simulink model "FluxModel2015a_verify_Q_zhixin"  (R2020b)
settings: Solver=VariableStepAuto  StartTime=0.0  StopTime=0.3  FixedStep=Ts  RelTol=1e-3  EnableMultiTasking=on
model workspace (MAT data in the model file):
  MOVE = Simulink.Parameter
  MOVE.Value = 1
  MOVE.DataType = 'boolean'
  MOVE.Dimensions = [1 1]
  STOP = Simulink.Parameter
  STOP.Value = 0
  STOP.DataType = 'boolean'
  STOP.Dimensions = [1 1]
  thres = Simulink.Parameter
  thres.Value = 0.1
  thres.DataType = 'double'
  thres.Dimensions = [1 1]
values from neighbouring files (symbols this model uses):
  AngleEncoderEn = 1    [parameters.m]
  AngleSpdClosedLoopEnable = 0.0    (= 0)    [parameters.m]
  CurrentLoopMax = Q14*1.2    (= 19660.8)    [parameters.m]
  EstOutMax_Speed_Q = Q14*1.2    (= 19660.8)    [parameters.m]
  Factor1 = Q15*Ts*Rb/Lq_realvalue    [parameters.m]
  Factor2 = Q15*Ts*Rs_realvalue/Lq_realvalue    (= 16990.2962963)    [parameters.m]
  fieldweaken_Max = 0    [parameters.m]
  fieldweaken_Min = -0.5*Q14    (= -8192)    [parameters.m]
  FieldWeakenEn = 0    [parameters.m]
  fluxF = Lam_realvalue/fluxB    [parameters.m]
  fluxF_Q14 = Q14*fluxF    [parameters.m]
  Friction = 0.003    [parameters.m]
  Ib = sqrt(2)*In    [parameters.m]
  Id_Ki = Q14*CurrentLoopBandwidth*Rs    [parameters.m]
  Id_Kp = Q14*CurrentLoopBandwidth*Ld    [parameters.m]
  IFCurrDecreased = 1    [parameters.m]
  IFCurrStart = 8    [parameters.m]
  IFCurrTarget = 5    [parameters.m]
  IFIdref = 0    [parameters.m]
  initial_degree = 0    [parameters.m]
  Iq_Ki = Q14*CurrentLoopBandwidth*Rs    [parameters.m]
  Iq_Kp = Q14*CurrentLoopBandwidth*Lq    [parameters.m]
  J_realvalue = 2.47e-4    (= 0.000247)    [parameters.m]
  KI_fieldweaken = 0.1*Q14    (= 1638.4)    [parameters.m]
  KP_fieldweaken = 1.0*Q14    (= 16384)    [parameters.m]
  LamObserverGain_Q = Q15*LamObserverGain    (= 13106.8)    [parameters.m]
  Ld = Ld_realvalue/Lb    [parameters.m]
  Ld_Q14 = Q14*Ld_realvalue/Lb    [parameters.m]
  Ld_realvalue = 2.7e-3    (= 0.0027)    [parameters.m]
  LowPassFilterBandWidth_Emf_Q = Q14*LowPassFilterBandWidth_Emf    (= 1445.64705882)    [parameters.m]
  LowPassFilterCoeff_Emf = Q15*(1/(1+LowPassFilterBandWidth_Emf*TsPu))    (= 31292.3812732)    [parameters.m]
  LowPassFilterCoeff_Spd = Q15*(1/(1+LowPassFilterBandWidth_Speed*SpeedloopTs/tb))    (= 20123.2126159)    [parameters.m]
  Lq = Lq_realvalue/Lb    [parameters.m]
  Lq_Q14 = Q14*Lq_realvalue/Lb    [parameters.m]
  Lq_realvalue = 2.7e-3    (= 0.0027)    [parameters.m]
  MOVE = 1    [parameters.m]
  Np = 1    [parameters.m]
  Omega0_Q = Q14*Omega0    (= 6553.6)    [parameters.m]
  OverModulationEn = 0    [parameters.m]
  PLL_KI = Q14*PLL_Bandwidth*PLL_Bandwidth    (= 56.6920415225)    [parameters.m]
  PLL_KP = Q14*2*PLL_Bandwidth    (= 1927.52941176)    [parameters.m]
  PLL_OUTMax_W = Q14*1.2    (= 19660.8)    [parameters.m]
  PWM_Period = 1000    [parameters.m]
  Q14 = 16384    [parameters.m]
  Q15 = 32767    [parameters.m]
  Q16 = 65535    [parameters.m]
  Rs = Rs_realvalue/Rb    [parameters.m]
  Rs_Q14 = Q14*Rs_realvalue/Rb    [parameters.m]
  Rs_realvalue = 28    [parameters.m]
  SecondOverMod = 0    [parameters.m]
  SMO_Gain = Q14*0.85    (= 13926.4)    [parameters.m]
  SMO_I_ERROR = Q14*0.05    (= 819.2)    [parameters.m]
  SpdClosedLoopEnable = 0.0    (= 0)    [parameters.m]
  Speed_Ki = Q14*SpeedLoopBandwidth    (= 481.882352941)    [parameters.m]
  Speed_Kp = Q14*SpeedLoopBandwidth*JPu/fluxF    [parameters.m]
  SpeedIncreased = 0.1*Wb    (= 1068.14150222)    [parameters.m]
  SpeedloopTs = 1/SpeedloopFrequency    (= 0.001)    [parameters.m]
  Speedn = 60*fn/Np    (= 102000)    [parameters.m]
  SpeedOutmax = 1.2*Q14    (= 19660.8)    [parameters.m]
  SpeedSwitch = 0.6*Wb    (= 6408.84901332)    [parameters.m]
  SpeedTarget = 0.8*Wb    (= 8545.13201776)    [parameters.m]
  STOP = 0    [parameters.m]
  SVCM_GAIN_Q = Q15*SVCM_GAIN    (= 26213.6)    [parameters.m]
  tb = 1/Wb    (= 9.36205547599e-05)    [parameters.m]
  Tf = 0    [parameters.m]
  thres = 0.1    [parameters.m]
  Tn = 0.012    [parameters.m]
  Ts = 1/SwitchFrequency    (= 5e-05)    [parameters.m]
  TsPu = Ts/tb    (= 0.53407075111)    [parameters.m]
  Vb = Vdc/sqrt(3)    [parameters.m]
  Vdc = sqrt(2)*Un    [parameters.m]
  Wb = 2*pi*fn    (= 10681.4150222)    [parameters.m]
  ZeroSeqInjectEn = 0.0    (= 0)    [parameters.m]
undefined symbols (not defined in the file or in its folder): DiscIntNeverNeededParam, EstOutMax_Theta, magnitude, sigbuilder_block
libraries: simulink x9, powerlib x5, mcbutilslib x1
(part 1 of 3)
settings Model: OrderedModelArguments=off  Creator=Administrator  LastModifiedBy=wangdi
settings DataIOCC: LimitDataPoints=on  SaveFormat=Array  ReturnWorkspaceOutputs=off
settings OptimizationCC: DefaultParameterBehavior=Inlined  DefaultUnderspecifiedDataType=single  EnhancedBackFolding=on  PassReuseOutputArgsAs=Individual arguments  ExpressionDepthLimit=2147483647  ZeroExternalMemoryAtStartup=off  ZeroInternalMemoryAtStartup=off  InitFltsAndDblsToZero=on  OptimizeBlockOrder=speed  DifferentSizesBufferReuse=on  OptimizationCustomize=off  EfficientTunableParamExpr=on
settings DebuggingCC: SaveWithParameterizedLinksMsg=none  UnderspecifiedInitializationDetection=Classic  MergeDetectMultiDrivingBlocksExec=none  SolverPrmCheckMsg=warning  ParameterTunabilityLossMsg=error  FcnCallInpInsideContextMsg=warning  StateNameClashWarn=warning  SFUnexpectedBacktrackingDiag=warning  SFNoUnconditionalDefaultTransitionDiag=warning  SFExecutionAtInitializationDiag=none  ArithmeticOperatorsInVariantConditions=warning
settings HardwareCC: ProdBitPerPointer=32  ProdBitPerSizeT=32  ProdBitPerPtrDiffT=32  ProdLargestAtomicFloat=None  ProdIntDivRoundTo=Undefined  ProdEndianess=Unspecified  ProdWordSize=32  ProdHWDeviceType=32-bit Generic
settings ModelReferenceCC: PropagateSignalLabelsOutOfModel=off
settings SFSimCC: SimUseLocalCustomCode=off  SimParseCustomCode=off  MATLABDynamicMemAlloc=off  CustomCodeUndefinedFunction=UseInterfaceOnly
settings RTWCC: Description=Embedded Coder  SystemTargetFile=ert.tlc  TemplateMakefile=ert_default_tmf  RTWUseLocalCustomCode=off
settings CodeAppCC: ForceParamTrailComments=on  IgnoreCustomStorageClasses=off  OperatorAnnotations=on  SimulinkDataObjDesc=on  SFDataObjDesc=on  InsertBlockDesc=on
settings ERTTargetCC: GenerateSampleERTMain=on  InlinedParameterPlacement=NonHierarchical  ERTCustomFileTemplate=example_file_process.tlc
settings ConfigComp: CovMetricSettings=dw  CovSaveCumulativeToWorkspaceVar=on  CovSaveSingleToWorkspaceVar=on  CovExternalEMLEnable=off
settings SimscapeCC: SimscapeNormalizeSystem=off

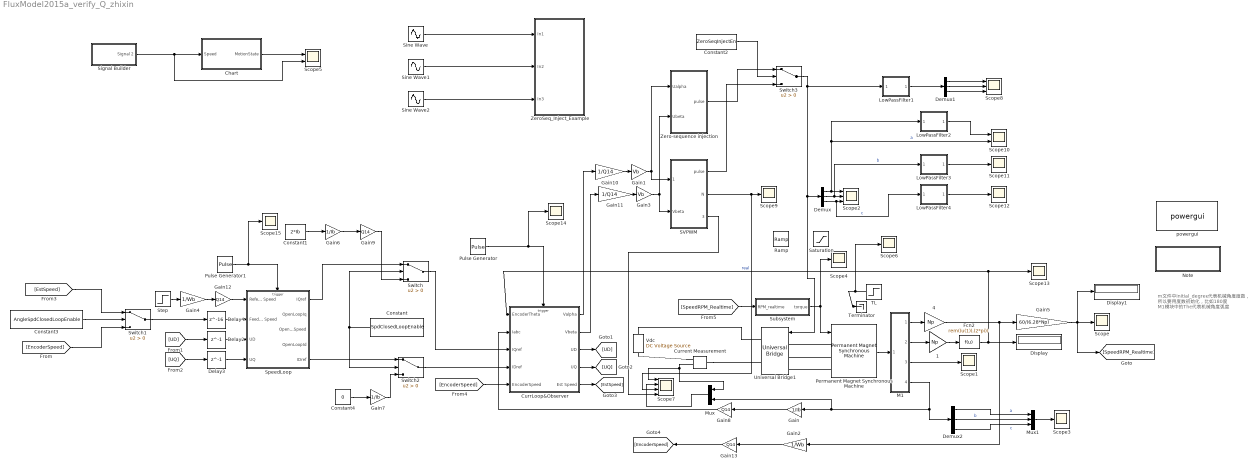
== system FluxModel2015a_verify_Q_zhixin ==
  note: m文件中initial_degree代表机械角度度数，
      | 所以要用度数初始化，比如180度
      | M1模块中的The代表机械角度弧度
  1 : Gain  Gain=Np
  4 : Gain  Gain=Np
  Chart : Stateflow chart  TreatAsAtomicUnit=on
  Constant : Constant  Value=SpdClosedLoopEnable
  Constant1 : Constant  Value=2*Ib
  Constant2 : Constant  Value=ZeroSeqInjectEn
  Constant3 : Constant  Value=AngleSpdClosedLoopEnable
  Constant4 : Constant  Value=0
  CurrLoop&Observer : Subsystem
  Current Measurement : powerlib/Measurements/Current Measurement  PhasorSimulation=off  OutputType=Complex  PSBequivalent=0
  Delay2 : Delay  DelayLength=1
  Delay3 : Delay  DelayLength=1
  Delay4 : Delay  DelayLength=16
  Demux : Demux  Outputs=3
  Demux1 : Demux  Outputs=3
  Demux2 : Demux  Outputs=3
  Display : Display
  Display1 : Display
  Fcn2 : Fcn  Expr=rem((u(1)),(2*pi))
  Gain : Gain  Gain=1/Ib
  Gain1 : Gain  Gain=Vb
  Gain10 : Gain  Gain=1/Q14
  Gain11 : Gain  Gain=1/Q14
  Gain{8..9,12..13} (4 alike) : Gain  Gain=Q14
  Gain2 : Gain  Gain=1/Wb
  Gain3 : Gain  Gain=Vb
  Gain4 : Gain  Gain=1/Wb
  Gain5 : Gain  Gain=60/(6.28*Np)
  Gain6 : Gain  Gain=1/Ib
  Gain7 : Gain  Gain=1/Ib
  LowPassFilter1 : Subsystem
  LowPassFilter2 : Subsystem
  LowPassFilter3 : Subsystem
  LowPassFilter4 : Subsystem
  M1 : Subsystem
  Mux : Mux  Inputs=2
  Mux1 : Mux  Inputs=3
  Note : Subsystem
  Permanent Magnet Synchronous Machine : powerlib/Machines/Permanent Magnet Synchronous Machine  NbPhases=3  FluxDistribution=Sinusoidal  RotorType=Salient-pole  MechanicalLoad=Torque Tm  PresetModel=No  ShowDetailedParameters=on  MeasurementBus=off  Resistance=Rs_realvalue  Inductance=8.5e-3  dqInductances=[Ld_realvalue, Lq_realvalue]  La=0.000835  MachineConstant=Flux linkage established by magnets (V.s)  Flux=Lam_realvalue  VoltageCst=11.7365  TorqueCst=0.09706  Flat=120  Mechanical=[J_realvalue Friction Np Tf]  PolePairs=Np  InitialConditions=[0,initial_degree, 0,0]  InitialConditions5ph=[0 0 0 0 0 0]  RefAngle=Aligned with phase A axis (original Park)  IterativeDiscreteModel=Trapezoidal non iterative  TsBlock=-1  TsPowergui=0
  Pulse Generator : DiscretePulseGenerator  PulseType=Time based  Period=Ts  PulseWidth=50
  Pulse Generator1 : DiscretePulseGenerator  PulseType=Time based  Period=SpeedloopTs  PulseWidth=50
  Ramp : simulink/Sources/Ramp  slope=5  start=0  InitialOutput=0
  SVPWM : Subsystem
  Saturation : Saturate  UpperLimit=0.2  LowerLimit=-0.2
  Scope{,1,3..4,6,9,11..15} (11 alike) : Scope
  Scope10 : Scope  NumInputPorts=2
  Scope2 : Scope  NumInputPorts=3
  Scope5 : Scope  NumInputPorts=2
  Scope7 : Scope  NumInputPorts=4
  Scope8 : Scope  NumInputPorts=3
  Signal Builder : Subsystem  Tag=STV Subsys  LoadFcn=sigbuilder_block('load');  StartFcn=sigbuilder_block('start');  StopFcn=sigbuilder_block('stop');  ClipboardFcn=sigbuilder_block('clipboard');  mask(Sigbuilder block){tuvar=[0:10]}
      mask help: Simulink:masks:SigbuilderBlock_MD
      mask init:
      | if ~strcmp(get_param(bdroot(gcbh),'SimulationStatus'),'stopped') tuvar = sigbuilder_block('maskInit'); end
      settings: CopyFcn=sigbuilder_block('copy');  DeleteFcn=sigbuilder_block('delete');  ModelCloseFcn=sigbuilder_block('modelClose');  PreSaveFcn=sigbuilder_block('preSave');  PauseFcn=sigbuilder_block('pause');  ContinueFcn=sigbuilder_block('continue');  NameChangeFcn=sigbuilder_block('namechange');  OpenFcn=sigbuilder_block('open',[1951.5 -31.5 550.5 326 ]);  CloseFcn=sigbuilder_block('close');
      mask Display: plot(0, 0, 100, 100,[2, 2, 32, 32, 2], [68, 8, 8, 68, 68],[32, 2], [38, 38], [32, 19, 2],[53, 60, 44], [32, 17, 17, 2],[16, 16, 31, 31]);txt = getActiveGroup(gcbh);text(2, 100, txt,'verticalAlignment', 'top');
  Sine Wave : Sin  Frequency=10*6.28
  Sine Wave1 : Sin  Frequency=10*6.28  Phase=2*pi/3
  Sine Wave2 : Sin  Frequency=10*6.28  Phase=4*pi/3
  SpeedLoop : Subsystem
  Step : Step  Time=0  After=1.5*Wb  SampleTime=0
  Subsystem : Subsystem
  Switch{,1..3} (4 alike) : Switch  Criteria=u2 > Threshold
  TL : Step  Time=0  Before=1  After=2.88  SampleTime=0
  Terminator : Terminator
  Universal Bridge1 : powerlib/Power Electronics/Universal Bridge  Arms=3  SnubberResistance=1e5  SnubberCapacitance=inf  Device=IGBT / Diodes  Ron=1e-3  Lon=0  ForwardVoltages="[  0  0  ]"  ForwardVoltage=0  GTOparameters=[ 10e-6 , 20e-6 ]  IGBTparameters=[ 1e-6 , 2e-6 ]  Measurements=None  Measurements_2=None  converterType=Rectifier
  Vdc : powerlib/Electrical Sources/DC Voltage Source  Amplitude=Vdc  Measurements=None
  Zero-sequence injection : Subsystem
  ZeroSeq_Inject_Example : Subsystem
  powergui : powerlib/powergui  SimulationMode=Discrete  SampleTime=Ts/100  frequency=60  Iterations=50  frequencyindice=0  Pbase=100e6  ErrMax=1e-4  UnitsV=kV  UnitsW=MW  buscounter=0  FunctionMessages=off  echomessages=off  EnableUseOfTLC=off  CurrentSourceSwitches=off  DisableSnubberDevices=off  DisableRonSwitches=off  DisableVfSwitches=off  DisplayEquations=off  AutomaticDiscreteSolvers=off  SolverType=Tustin/Backward Euler (TBE)  Interpol=off  ExternalGateDelay=off  methode=off  Ts=0  x0status=blocks  SPID=off  SwTol=0  HookPort=off  NonlinearTolerance=1e-4  nMaxIteration=100  ContinueOnMaxIteration=off  RestoreLinks=warning  ResistiveCurrentMeasurement=off  Frange=[0:2:500]  Ylog=off  Xlog=on  ShowGrid=off  save=off  variable=ZData  structure=0  ZoomFFT=off  StartTime=0.0  cycles=1  DisplayStyle=1  fundamental=60  FreqAxis=off  MaxFrequency=1000  frequencyindicesteady=1  RmsSteady=1  display=off
  wires:
  M1/4(Iabc) -> Demux2/1, Mux/2, Gain/1
  M1/2(The) -> 1/1
  Permanent Magnet Synchronous Machine/1 -> M1/1(In1)
  1/1 -> Fcn2/1
  M1/1(wm) -> 4/1
  M1/3(Te) -> Scope1/1
  4/1 -> Gain5/1, Gain2/1
  Fcn2/1 -> Display/1, CurrLoop&Observer/1(EncoderTheta), Scope13/1  "real"
  Pulse Generator/1 -> Scope14/1, CurrLoop&Observer/Trigger
  Demux2/1 -> Mux1/1  "a"
  Demux2/2 -> Mux1/2  "b"
  Demux2/3 -> Mux1/3  "c"
  Demux/1 -> Scope10/2, LowPassFilter2/1(Input), Scope2/1  "a"
  Demux/2 -> LowPassFilter3/1(Input), Scope2/2  "b"
  Demux/3 -> LowPassFilter4/1(Input), Scope2/3  "c"
  TL/1 -> Scope6/1, Terminator/1
  Gain/1 -> Gain8/1
  Current Measurement/1 -> Mux/1, Scope7/1
  Mux/1 -> Scope7/2
  SVPWM/2(N) -> Scope7/3, Scope9/1
  SVPWM/3(Output) -> Scope7/4
  LowPassFilter1/1(Output) -> Demux1/1
  Demux1/1 -> Scope8/1
  Demux1/2 -> Scope8/2
  Demux1/3 -> Scope8/3
  LowPassFilter2/1(Output) -> Scope10/1
  LowPassFilter3/1(Output) -> Scope11/1
  LowPassFilter4/1(Output) -> Scope12/1
  Mux1/1 -> Scope3/1
  Gain5/1 -> [SpeedRPM_Realtime], Display1/1, Scope/1
  Pulse Generator1/1 -> Scope15/1, SpeedLoop/Trigger
  Gain6/1 -> Gain9/1
  Constant1/1 -> Gain6/1
  CurrLoop&Observer/3(UD) -> [UD]
  CurrLoop&Observer/4(UQ) -> [UQ]
  [UD] -> Delay2/1
  [UQ] -> Delay3/1
  SpeedLoop/1(IQref) -> Switch/1
  Step/1 -> Gain4/1
  CurrLoop&Observer/5(Est Speed) -> [EstSpeed]
  Constant3/1 -> Switch1/2
  [EstSpeed] -> Switch1/1
  [EncoderSpeed] -> Switch1/3
  [EncoderSpeed] -> CurrLoop&Observer/5(EncoderSpeed)
  Delay2/1 -> SpeedLoop/3(UD)
  Delay3/1 -> SpeedLoop/4(UQ)
  Delay4/1 -> SpeedLoop/2(Feedback Speed)
  Signal Builder/1(Signal 2) -> Scope5/2, Chart/1(Speed)
  Chart/1(MotionState) -> Scope5/1
  Constant/1 -> Switch2/2, Switch/2
  Constant4/1 -> Gain7/1
  Gain7/1 -> Switch2/3
  Gain8/1 -> CurrLoop&Observer/2(Iabc)
  Gain9/1 -> Switch/3
  Gain10/1 -> Gain1/1
  Gain11/1 -> Gain3/1
  Gain4/1 -> Gain12/1
  Gain2/1 -> Gain13/1
  Switch/1 -> CurrLoop&Observer/3(IQref)
  Switch2/1 -> CurrLoop&Observer/4(IDref)
  Switch1/1 -> Delay4/1
  Gain12/1 -> SpeedLoop/1(Reference Speed)
  Gain13/1 -> [EncoderSpeed]
  SpeedLoop/5(IDref) -> Switch2/1
  CurrLoop&Observer/1(Valpha) -> Gain10/1
  CurrLoop&Observer/2(Vbeta) -> Gain11/1
  Subsystem/1(torque) -> Permanent Magnet Synchronous Machine/1, Scope4/1
  [SpeedRPM_Realtime] -> Subsystem/1(RPM_realtime)
  Gain1/1 -> Zero-sequence injection/1(Ualpha), SVPWM/1(Valpha)
  Gain3/1 -> SVPWM/2(Vbeta), Zero-sequence injection/2(Ubeta)
  Constant2/1 -> Switch3/2
  Zero-sequence injection/1(pulse) -> Switch3/1
  SVPWM/1(pulse) -> Switch3/3
  Switch3/1 -> Demux/1, Universal Bridge1/1, LowPassFilter1/1(Input)
  Sine Wave/1 -> ZeroSeq_Inject_Example/1(In1)
  Sine Wave1/1 -> ZeroSeq_Inject_Example/2(In2)
  Sine Wave2/1 -> ZeroSeq_Inject_Example/3(In3)
  connections:
  Permanent Magnet Synchronous Machine/LConn3 -- Universal Bridge1/LConn3
  Vdc/RConn1 -- Universal Bridge1/RConn1
  Permanent Magnet Synchronous Machine/LConn1 -- Universal Bridge1/LConn1
  Permanent Magnet Synchronous Machine/LConn2 -- Universal Bridge1/LConn2
  Current Measurement/LConn1 -- Universal Bridge1/RConn2
  Current Measurement/RConn1 -- Vdc/LConn1

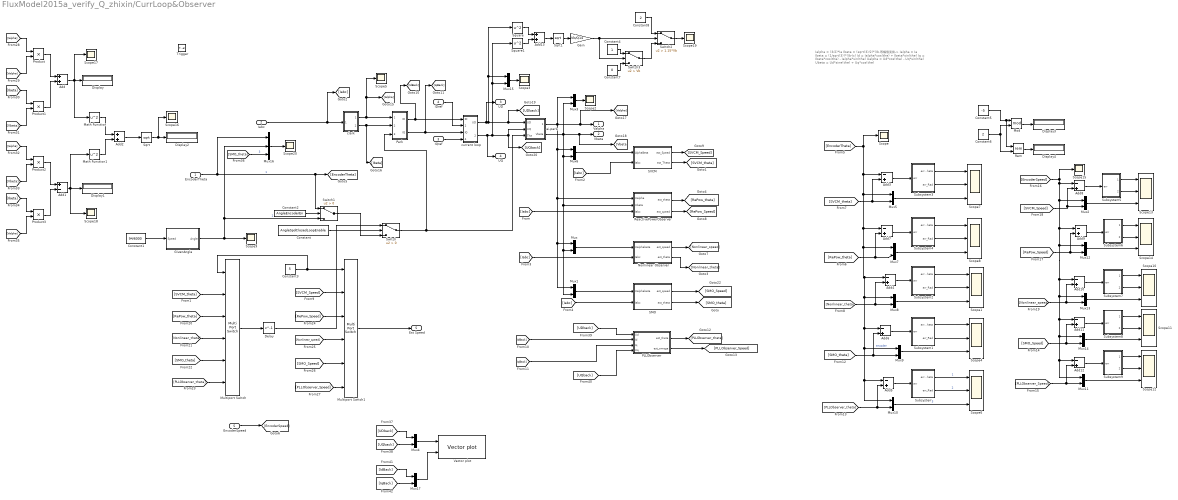
== system FluxModel2015a_verify_Q_zhixin/CurrLoop&Observer ==
  note: Ialpha = (3/2)*Ia
      | Ibeta = (sqrt(3)/2)*(Ib-Ic)
      | 等幅值变换->
      | Ialpha = Ia
      | Ibeta = (1/sqrt(3))*(Ib-Ic)
      |
      | Id = Ialpha*cos(the) + Ibeta*sin(the)
      | Iq = Ibeta*cos(the) - Ialpha*sin(the)
      |
      | Ualpha = Ud*cos(the) - Uq*sin(the)
      | Ubeta = Ud*sine(the) + Uq*cos(the)
  EncoderTheta : Inport
  Iabc : Inport  Port=2
  IQref : Inport  Port=3
  IDref : Inport  Port=4
  EncoderSpeed : Inport  Port=5
  Trigger : TriggerPort  VariantControl=(inherit)
  Add : Sum
  Add1 : Sum  Inputs=+-
  Add{3..12} (10 alike) : Sum  Inputs=-+
  Add13 : Sum
  Add2 : Sum
  Constant : Constant  Value=AngleSpdClosedLoopEnable
  Constant1 : Constant  Value=94/6000
  Constant2 : Constant  Value=AngleEncoderEn
  Constant3 : Constant  Value=5
  Constant4 : Constant
  Constant5 : Constant  Value=-5
  Constant6 : Constant  Value=2
  Constant7 : Constant  Value=0
  Constant8 : Constant  Value=2
  Delay : Delay  DelayLength=1
  Display{,1..4} (5 alike) : Display
  Gain : Gain  Gain=Vb/Q14
  GivenAngle : Subsystem
  Math Function : Math  Operator=square  SaturateOnIntegerOverflow=on
  Math Function1 : Math  Operator=square  SaturateOnIntegerOverflow=on
  Mod : Math  Operator=mod  SaturateOnIntegerOverflow=on
  Multiport Switch : MultiPortSwitch  Inputs=5
  Multiport Switch1 : MultiPortSwitch  Inputs=5
  Mux{,1..15,17} (17 alike) : Mux  Inputs=2
  Mux16 : Mux  Inputs=3
  Nonlinear Observer : Subsystem
  PLLObserver : Subsystem
  Park : Subsystem
  Product{,1..3} (4 alike) : Product
  ReactivePowerObserver : Subsystem
  Rem : Math  Operator=rem  SaturateOnIntegerOverflow=on
  SMO : Subsystem
  SVCM : Subsystem
  Scope{,2..3,5,9,15..20} (11 alike) : Scope
  Scope{1,4,6..8,10..14} (10 alike) : Scope  NumInputPorts=3
  Sqrt : Sqrt  SaturateOnIntegerOverflow=on
  Sqrt1 : Sqrt  SaturateOnIntegerOverflow=on
  Square : Math  Operator=square  SaturateOnIntegerOverflow=on
  Square1 : Math  Operator=square  SaturateOnIntegerOverflow=on
  Subsystem : Subsystem
  Subsystem1 : Subsystem
  Subsystem2 : Subsystem
  Subsystem3 : Subsystem
  Subsystem4 : Subsystem
  Subsystem5 : Subsystem
  Subsystem6 : Subsystem
  Subsystem7 : Subsystem
  Subsystem8 : Subsystem
  Subsystem9 : Subsystem
  Switch : Switch  Criteria=u2 > Threshold
  Switch1 : Switch  Criteria=u2 > Threshold
  Switch2 : Switch  Criteria=u2 > Threshold  Threshold=1.15*Vb
  Switch3 : Switch  Criteria=u2 > Threshold  Threshold=Vb
  Vector plot : mcbutilslib/Vector plot  InputSignals=Vdq Idq  ReferenceFrame=Rotating Reference Frame  axisAlign=D-axis  thetaUnits=Radians  angleUnits=Radians  OpenFigAtSimStart=on  debugEnable=0
      settings: SourceProductBaseCode=MT
  ai-park : Subsystem
  clark : Subsystem
  current loop : Subsystem
  Valpha : Outport
  Vbeta : Outport  Port=2
  UD : Outport  Port=3
  UQ : Outport  Port=4
  Est Speed : Outport  Port=5
  wires:
  Iabc/1 -> [Iabc], clark/1(Iabc)
  Park/1(ID) -> current loop/1(ID), [IdBack]
  Park/2(IQ) -> current loop/3(IQ), [IqBack]
  Mux3/1 -> Scope2/1
  EncoderTheta/1 -> Mux16/1, Switch1/1, [EncoderTheta]  "1"
  ai-park/1(Valpha) -> Mux3/1, ReactivePowerObserver/1(Ualpha), Mux1/1, Mux/1, Mux6/1, [Valpha], Valpha/1
  ai-park/2(Vbeta) -> Mux3/2, ReactivePowerObserver/2(Ubeta), Mux1/2, Mux/2, Mux6/2, [Vbeta], Vbeta/1
  [Iabc] -> ReactivePowerObserver/3(Iabc)
  Mux/1 -> Nonlinear Observer/1(Ualphabeta)
  [Iabc] -> Nonlinear Observer/2(Iabc)
  Nonlinear Observer/2(est_theta) -> [Nonlinear_theta]
  ReactivePowerObserver/1(est_theta) -> [RePow_theta]
  Mux1/1 -> SMO/1(Ualphabeta)
  [Iabc] -> SMO/2(Iabc)
  Mux7/1 -> Scope8/3
  Nonlinear Observer/1(est_speed) -> [Nonlinear_speed]
  ReactivePowerObserver/2(est_speed) -> [RePow_Speed]
  clark/1(Ialpha) -> Scope5/1, [Ialpha], Park/1(alpha)
  clark/2(Ibeta) -> [Ibeta], Park/2(beta)
  [IdBack] -> PLLObserver/2(Id)
  [IqBack] -> PLLObserver/3(Iq)
  [PLLObserver_theta] -> Add5/2, Mux10/2
  [EncoderSpeed] -> Scope15/1, Add8/1, Mux2/1, Add10/1, Mux13/1, Add11/1, Mux14/1, Mux11/1, Add12/1, Mux12/1, Add9/1
  [SVCM_theta] -> Multiport Switch/2
  [RePow_theta] -> Multiport Switch/3
  [Nonlinear_theta] -> Multiport Switch/4
  [SMO_theta] -> Multiport Switch/5
  [PLLObserver_theta] -> Multiport Switch/6
  Constant3/1 -> Multiport Switch/1, Multiport Switch1/1
  [SVCM_Speed] -> Multiport Switch1/2
  [RePow_Speed] -> Multiport Switch1/3
  [Nonlinear_speed] -> Multiport Switch1/4
  [SMO_Speed] -> Multiport Switch1/5
  [PLLObserver_Speed] -> Multiport Switch1/6
  [Ialpha] -> Product/1
  [Valpha] -> Product/2
  [Vbeta] -> Product1/2
  [Ibeta] -> Product1/1
  Product/1 -> Add/1
  Product1/1 -> Add/2
  Add/1 -> Scope17/1, Math Function/1, Display/1
  Add1/1 -> Scope18/1, Math Function1/1, Display1/1
  Product3/1 -> Add1/2
  Product2/1 -> Add1/1
  [Ibeta] -> Product3/1
  [Valpha] -> Product3/2
  [Vbeta] -> Product2/2
  [Ialpha] -> Product2/1
  Math Function/1 -> Add2/1
  Math Function1/1 -> Add2/2
  Add2/1 -> Sqrt/1
  Sqrt/1 -> Scope16/1, Display2/1
  IDref/1 -> current loop/2(IDref)
  IQref/1 -> current loop/4(IQref)
  [SMO_theta] -> Mux9/2, Add6/2
  [EncoderTheta] -> Add3/1, Mux5/1, Add7/1, Mux8/1, Add6/1, Mux9/1, Add5/1, Mux10/1, Add4/1, Mux7/1, Scope/1  "encoder"
  SMO/1(est_speed) -> [SMO_Speed]
  SMO/2(est_theta) -> [SMO_theta]
  Constant5/1 -> Rem/1, Mod/1
  Constant6/1 -> Mod/2, Rem/2
  Mod/1 -> Display3/1
  Rem/1 -> Display4/1
  Add5/1 -> Subsystem/1(err)
  Subsystem/1(err_Theta) -> Scope6/1  "1"
  Subsystem/2(err_Rad) -> Scope6/2  "2"
  Mux10/1 -> Scope6/3  "3"
  Add6/1 -> Subsystem1/1(err)
  Subsystem1/1(err_Theta) -> Scope4/1
  Subsystem1/2(err_Rad) -> Scope4/2
  Add4/1 -> Subsystem2/1(err)
  Subsystem2/1(err_Theta) -> Scope1/1
  Subsystem2/2(err_Rad) -> Scope1/2
  Mux8/1 -> Scope1/3
  [Nonlinear_theta] -> Add4/2, Mux8/2
  Add3/1 -> Subsystem3/1(err)
  Subsystem3/1(err_Theta) -> Scope7/1
  Subsystem3/2(err_Rad) -> Scope7/2
  Mux5/1 -> Scope7/3
  [SVCM_theta] -> Add3/2, Mux5/2
  Add7/1 -> Subsystem4/1(err)
  Subsystem4/1(err_Theta) -> Scope8/1
  Subsystem4/2(err_Rad) -> Scope8/2
  [RePow_theta] -> Add7/2, Mux7/2
  Add8/1 -> Subsystem5/1(err)
  Subsystem5/1(err_Spd) -> Scope13/1
  Subsystem5/2(err_Fhz) -> Scope13/2
  Mux2/1 -> Scope13/3
  [SVCM_Speed] -> Add8/2, Mux2/2
  Add9/1 -> Subsystem6/1(err)
  Subsystem6/1(err_Spd) -> Scope14/1
  Subsystem6/2(err_Fhz) -> Scope14/2
  Mux12/1 -> Scope14/3
  [RePow_Speed] -> Add9/2, Mux12/2
  Add10/1 -> Subsystem7/1(err)
  Subsystem7/1(err_Spd) -> Scope10/1
  Subsystem7/2(err_Fhz) -> Scope10/2
  Mux13/1 -> Scope10/3
  [Nonlinear_speed] -> Add10/2, Mux13/2
  Add11/1 -> Subsystem8/1(err)
  Subsystem8/1(err_Spd) -> Scope11/1
  Subsystem8/2(err_Fhz) -> Scope11/2
  Mux14/1 -> Scope11/3
  [SMO_Speed] -> Add11/2, Mux14/2
  Add12/1 -> Subsystem9/1(err)
  Subsystem9/1(err_Spd) -> Scope12/1
  Subsystem9/2(err_Fhz) -> Scope12/2
  Mux11/1 -> Scope12/3
  [PLLObserver_Speed] -> Add12/2, Mux11/2
  PLLObserver/1(est_theta) -> [PLLObserver_theta]
  PLLObserver/2(est_omega) -> [PLLObserver_Speed]
  [UDback] -> PLLObserver/1(Ud)
  [UQback] -> PLLObserver/4(Uq)
  Multiport Switch1/1 -> Est Speed/1
  Constant/1 -> Switch/2
  EncoderSpeed/1 -> [EncoderSpeed]
  Constant1/1 -> GivenAngle/1(Speed)
  GivenAngle/1(Angle) -> Scope9/1, Switch1/3, Mux16/2  "2"
  Mux9/1 -> Scope4/3
  [SMO_theta] -> Mux16/3  "3"
  Mux16/1 -> Scope20/1
  Constant2/1 -> Switch1/2
  Switch1/1 -> Switch/3
  Multiport Switch/1 -> Delay/1
  Switch/1 -> Park/3(theta), ai-park/3(The)
  [Iabc] -> SVCM/2(Iabc)
  Mux6/1 -> SVCM/1(AlphaBeta)
  SVCM/1(est_Speed) -> [SVCM_Speed]
  SVCM/2(est_Theta) -> [SVCM_theta]
  Square/1 -> Add13/1
  Square1/1 -> Add13/2
  Add13/1 -> Sqrt1/1
  Sqrt1/1 -> Gain/1
  Switch2/1 -> Scope19/1
  Constant8/1 -> Switch2/1
  Switch3/1 -> Switch2/3
  Constant4/1 -> Switch3/1
  Constant7/1 -> Switch3/3
  Gain/1 -> Switch3/2, Switch2/2
  Delay/1 -> Switch/1
  current loop/1(UD) -> Square/1, Mux15/1, ai-park/1(UD), [UDback], UD/1
  current loop/2(UQ) -> Square1/1, Mux15/2, [UQback], ai-park/2(UQ), UQ/1
  Mux15/1 -> Scope3/1
  Mux4/1 -> Vector plot/1
  [UQback] -> Mux4/2
  [UDback] -> Mux4/1
  [IdBack] -> Mux17/1
  [IqBack] -> Mux17/2
  Mux17/1 -> Vector plot/2

== system FluxModel2015a_verify_Q_zhixin/LowPassFilter1 ==
  Input : Inport
  Add : Sum  Inputs=+-
  Add1 : Sum
  Constant : Constant
  Constant1 : Constant  Value=1/(1+20*Ts)
  Delay6 : Delay  DelayLength=1
  Gain : Gain  Gain=1/(1+20*Ts)
  Product : Product
  Output : Outport
  wires:
  Add1/1 -> Output/1, Delay6/1
  Gain/1 -> Add1/2
  Product/1 -> Add1/1
  Add/1 -> Product/2
  Input/1 -> Product/1
  Constant1/1 -> Add/2
  Constant/1 -> Add/1
  Delay6/1 -> Gain/1

== system FluxModel2015a_verify_Q_zhixin/LowPassFilter2 ==
  Input : Inport
  Add : Sum  Inputs=+-
  Add1 : Sum
  Constant : Constant
  Constant1 : Constant  Value=1/(1+20*Ts)
  Delay6 : Delay  DelayLength=1
  Gain : Gain  Gain=1/(1+20*Ts)
  Product : Product
  Output : Outport
  wires:
  Add1/1 -> Output/1, Delay6/1
  Gain/1 -> Add1/2
  Product/1 -> Add1/1
  Add/1 -> Product/2
  Input/1 -> Product/1
  Constant1/1 -> Add/2
  Constant/1 -> Add/1
  Delay6/1 -> Gain/1

== system FluxModel2015a_verify_Q_zhixin/LowPassFilter3 ==
  Input : Inport
  Add : Sum  Inputs=+-
  Add1 : Sum
  Constant : Constant
  Constant1 : Constant  Value=1/(1+20*Ts)
  Delay6 : Delay  DelayLength=1
  Gain : Gain  Gain=1/(1+20*Ts)
  Product : Product
  Output : Outport
  wires:
  Delay6/1 -> Gain/1
  Constant/1 -> Add/1
  Constant1/1 -> Add/2
  Input/1 -> Product/1
  Add/1 -> Product/2
  Product/1 -> Add1/1
  Gain/1 -> Add1/2
  Add1/1 -> Delay6/1, Output/1

== system FluxModel2015a_verify_Q_zhixin/LowPassFilter4 ==
  Input : Inport
  Add : Sum  Inputs=+-
  Add1 : Sum
  Constant : Constant
  Constant1 : Constant  Value=1/(1+20*Ts)
  Delay6 : Delay  DelayLength=1
  Gain : Gain  Gain=1/(1+20*Ts)
  Product : Product
  Output : Outport
  wires:
  Add1/1 -> Output/1, Delay6/1
  Gain/1 -> Add1/2
  Product/1 -> Add1/1
  Add/1 -> Product/2
  Input/1 -> Product/1
  Constant1/1 -> Add/2
  Constant/1 -> Add/1
  Delay6/1 -> Gain/1

== system FluxModel2015a_verify_Q_zhixin/M1 ==
  In1 : Inport
  Bus Selector : BusSelector  OutputSignals=Stator current is_a (A),Stator current is_b (A),Stator current is_c (A)
  Bus Selector1 : BusSelector  OutputSignals=Rotor speed wm (rad/s),Rotor angle thetam (rad),Electromagnetic torque Te (N*m)
  Mux : Mux  Inputs=3
  wm : Outport
  The : Outport  Port=2
  Te : Outport  Port=3
  Iabc : Outport  Port=4
  wires:
  Bus Selector/1 -> Mux/1  "<Stator current is_a (A)>"
  Bus Selector/2 -> Mux/2  "<Stator current is_b (A)>"
  Bus Selector/3 -> Mux/3  "<Stator current is_c (A)>"
  Bus Selector1/1 -> wm/1  "<Rotor speed wm (rad/s)>"
  Bus Selector1/2 -> The/1  "<Rotor angle thetam (rad)>"
  Bus Selector1/3 -> Te/1  "<Electromagnetic torque Te (N*m)>"
  Mux/1 -> Iabc/1
  In1/1 -> Bus Selector1/1, Bus Selector/1

== system FluxModel2015a_verify_Q_zhixin/Note ==
  note: 移位
  note: 按位与
  note: 多输入开关
  note: 双输入开关
  note: $1.定子三相电压方程：\\ u_a = R_s i_a + \frac{d\psi_a}{dt}\\ u_b = R_s i_b + \frac{d\psi_b}{dt}\\ u_c = R_s i_c + \frac{d\psi_c}{dt}$
  note: 3. 常用模块
  note: 单位延时：Unit Delay
  note: 2.刹车方式：
      | 	a. 短路刹车，若参与PWM抬升母线电压
      | 	b. Iq负电流刹车，抬升母线电压
      | 	c. Id正电流刹车，电机本体发热
  note: 1.30°以内Theta_rads近似Sin(Theta_rads)
  note: 单位延时：Repeating Sequence
  note: 斜坡函数：Ramp
  note: 限幅函数：Saturation
  note: 条件函数：Switch
  note: 积分函数：Discrete-Time Integrator
  note: 功能函数：MATLAB Function
  note: $2.两相静止坐标系电机方程\\ u_\alpha = R_s i_\alpha + L_\alpha\frac{di_\alpha}{dt}+L_{\alpha\beta}\frac{di_\beta}{dt}-\omega_e \psi_rsin(\theta)\\ u_\beta = R_s i_\beta + L_\beta\frac{di_\beta}{dt}+L_{\alpha\beta}\frac{di_\alpha}{dt}+\omega_e \psi_rsin(\theta)\\ L=\frac{1}{2}(L_d+L_q)\\ {\Delta}L=\frac{1}{2}(L_d-L_q)\\ L_\alpha = L + {\Delta}Lcos(2\theta)\\ L_\beta = L - {\Delta}Lcos(2\theta)\\ L_{\alpha\beta}= {\Delta}Lsin(2\theta)\\ \\ 有功功率：P=u_\alpha i_\alpha + u_\beta i_\beta\\ 无功功率：Q=u_\beta i_\alpha - u_\alpha i_\beta\\ 视在功率：S=\sqrt{P^2+Q^2}\\$
  note: $3.旋转坐标系电机方程\\ \psi_d =L_di_d+\psi_r\\ \psi_q=L_qi_q\\ u_d=R_si_d+\frac{d\psi_d}{dt}-\omega_e\psi_q\\ u_q=R_si_q+\frac{d\psi_q}{dt}+\omega_e\psi_d\\ u_d = R_s i_d + L_d\frac{di_d}{dt}-\omega_eL_qi_q\\ u_q = R_s i_q + L_q\frac{di_q}{dt}+\omega_eL_di_d+\omega_e\psi_r\\ \\ 有功功率：P=u_d i_d + u_q i_q\\ 无功功率：Q=u_q i_d - u_d i_q\\ 视在功率：S=\sqrt{P^2+Q^2}\\ 电磁转矩：T_e=\frac{3}{2}P_ni_q[i_d(L_d-L_q)+\psi_r]\\ SPM电磁转矩:T_e=\frac{3}{2}P_n\psi_ri_q$
  note: $运动方程：T_e-T_L=\frac{J}{N_p}\frac{d\omega}{dt}\\ 功率方程：P_t=T_e\omega_r\\ 功率因素：cos(\phi)=\frac{P}{Q}\\ 效率：\eta=\frac{P_t}{P}$
  Bitwise Operator : simulink/Logic and Bit Operations/Bitwise Operator  Commented=on  logicop=AND  UseBitMask=on  BitMask=bin2dec('11011001')  BitMaskRealWorld=Stored Integer
  Discrete-Time Integrator1 : DiscreteIntegrator  Commented=on  gainval=Ts  SampleTime=-1  ICPrevOutput=DiscIntNeverNeededParam  ICPrevScaledInput=DiscIntNeverNeededParam
  MATLAB Function : MATLAB Function  Commented=on  TreatAsAtomicUnit=on
  Manual Switch : ManualSwitch  Commented=on
  Multiport Switch : MultiPortSwitch  Commented=on
  Ramp : simulink/Sources/Ramp  Commented=on  slope=10  start=0  InitialOutput=0
  Ramp1 : simulink/Sources/Ramp  Commented=on  slope=1  start=0  InitialOutput=0
  Repeating Sequence : simulink/Sources/Repeating Sequence  Commented=on  rep_seq_t=[0 2]  rep_seq_y=[0 2]
  Saturation : Saturate  Commented=on  UpperLimit=pi/2  LowerLimit=-pi/2
  Saturation1 : Saturate  Commented=on  UpperLimit=1000  LowerLimit=0
  Scope10 : Scope  Commented=on  NumInputPorts=2
  Shift Arithmetic : ArithShift  Commented=on  BitShiftNumber=8
  Sin : Trigonometry  Commented=on
  Switch : Switch  Commented=on  Criteria=u2 > Threshold
  Unit Delay : UnitDelay  Commented=on  SampleTime=-1  HasFrameUpgradeWarning=on
  wires:
  Ramp/1 -> Saturation/1
  Sin/1 -> Scope10/1
  Saturation/1 -> Scope10/2, Sin/1

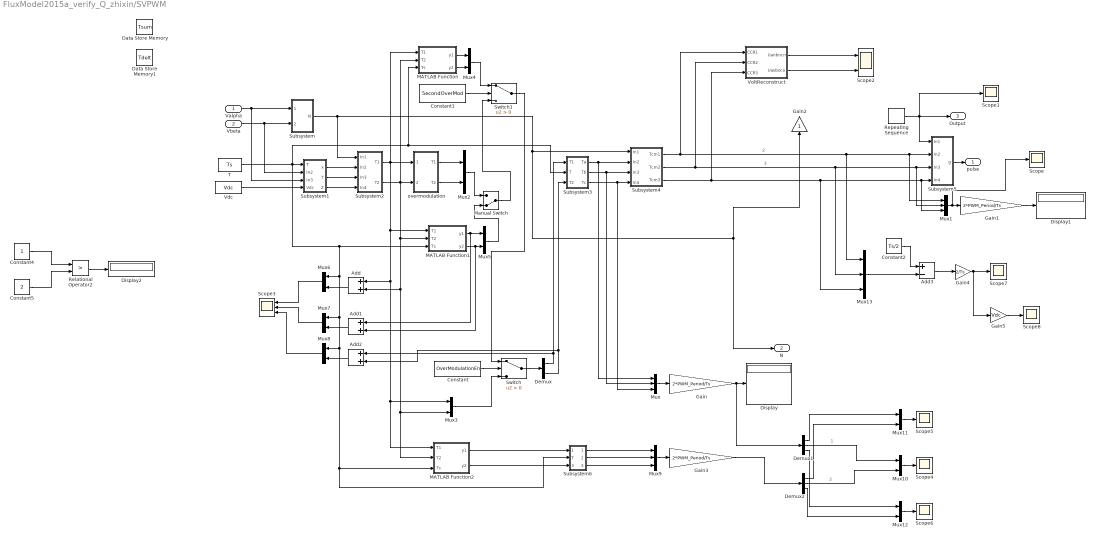
== system FluxModel2015a_verify_Q_zhixin/SVPWM ==
  Valpha : Inport
  Vbeta : Inport  Port=2
  Add : Sum
  Add1 : Sum
  Add2 : Sum
  Add3 : Sum  Inputs=+-
  Constant : Constant  Value=OverModulationEn
  Constant1 : Constant  Value=SecondOverMod
  Constant2 : Constant  Value=Ts/2
  Constant4 : Constant
  Constant5 : Constant  Value=2
  Data Store Memory : DataStoreMemory  DataStoreName=Tsum  ReadBeforeWriteMsg=warning  WriteAfterWriteMsg=warning  WriteAfterReadMsg=warning  ShowAdditionalParam=off  OutDataTypeStr=double
  Data Store Memory1 : DataStoreMemory  DataStoreName=Tdelt  ReadBeforeWriteMsg=warning  WriteAfterWriteMsg=warning  WriteAfterReadMsg=warning  ShowAdditionalParam=off  OutDataTypeStr=double
  Demux : Demux  Outputs=2
  Demux1 : Demux  Outputs=3
  Demux2 : Demux  Outputs=3
  Display : Display
      settings: Decimation=2
  Display1 : Display
      settings: Decimation=2
  Display2 : Display
  Gain : Gain  Gain=2*PWM_Period/Ts
  Gain1 : Gain  Gain=2*PWM_Period/Ts
  Gain2 : Gain
  Gain3 : Gain  Gain=2*PWM_Period/Ts
  Gain4 : Gain  Gain=2/Ts
  Gain5 : Gain  Gain=Vdc
  MATLAB Function : MATLAB Function  TreatAsAtomicUnit=on
  MATLAB Function1 : MATLAB Function  TreatAsAtomicUnit=on
  MATLAB Function2 : MATLAB Function  TreatAsAtomicUnit=on
  Manual Switch : ManualSwitch  CurrentSetting=0
  Mux{,1,9,13} (4 alike) : Mux  Inputs=3
  Mux{2..8,10..12} (10 alike) : Mux  Inputs=2
  Relational Operator2 : RelationalOperator  Operator=>  OutDataTypeStr=boolean  RndMeth=Simplest
  Repeating Sequence : simulink/Sources/Repeating Sequence  rep_seq_t=[0 Ts/2 Ts]  rep_seq_y=[0 Ts/2 0]
  Scope{,1,4..8} (7 alike) : Scope
  Scope2 : Scope  NumInputPorts=2
  Scope3 : Scope  NumInputPorts=3
  Subsystem : Subsystem
  Subsystem1 : Subsystem
  Subsystem2 : Subsystem
  Subsystem3 : Subsystem
  Subsystem4 : Subsystem
  Subsystem5 : Subsystem
  Subsystem6 : Subsystem
  Switch : Switch  Criteria=u2 > Threshold
  Switch1 : Switch  Criteria=u2 > Threshold
  T : Constant  Value=Ts
  Vdc : Constant  Value=Vdc
  VoltReconstruct : Subsystem
  overmodulation : Subsystem
  pulse : Outport
  N : Outport  Port=2
  Output : Outport  Port=3
  wires:
  Subsystem5/1(g) -> pulse/1
  Repeating Sequence/1 -> Scope1/1, Subsystem5/1(In1), Output/1
  Subsystem4/3(Tcm3) -> VoltReconstruct/3(CCR3), Mux13/3, Mux1/3, Subsystem5/4(In4)
  Subsystem4/2(Tcm2) -> VoltReconstruct/2(CCR2), Mux13/2, Mux1/2, Subsystem5/3(In3)  "3"
  Subsystem4/1(Tcm1) -> VoltReconstruct/1(CCR1), Mux13/1, Mux1/1, Subsystem5/2(In2)  "2"
  Subsystem3/3(Tc) -> Subsystem4/4(In4), Mux/3
  Subsystem3/2(Tb) -> Subsystem4/3(In3), Mux/2
  Subsystem3/1(Ta) -> Subsystem4/2(In2), Mux/1
  Subsystem1/3(Z) -> Subsystem2/4(In4)
  Subsystem1/2(Y) -> Subsystem2/3(In3)
  Subsystem1/1(x) -> Subsystem2/2(In2)
  Subsystem/1(N) -> Subsystem4/1(In1), Gain2/1, N/1, Subsystem2/1(In1)
  Vdc/1 -> Subsystem1/4(Vdc)
  Vbeta/1 -> Subsystem1/2(In2), Subsystem/2(Vbeta)
  Valpha/1 -> Subsystem1/3(In3), Subsystem/1(Valpha)
  Mux/1 -> Gain/1
  Gain/1 -> Demux1/1, Display/1
  Mux1/1 -> Scope/1, Gain1/1
  Gain1/1 -> Display1/1
  Constant4/1 -> Relational Operator2/1
  Constant5/1 -> Relational Operator2/2
  Relational Operator2/1 -> Display2/1
  Subsystem2/1(T1) -> MATLAB Function/1(T1), MATLAB Function1/1(T1), Add/1, MATLAB Function2/1(T1), Mux3/1, overmodulation/1(1)
  Subsystem2/2(T2) -> MATLAB Function/2(T2), overmodulation/2(2), MATLAB Function1/2(T2), MATLAB Function2/2(T2), Mux3/2, Add/2
  Constant/1 -> Switch/2
  overmodulation/1(T1) -> Mux2/1
  overmodulation/2(T2) -> Mux2/2
  Mux3/1 -> Switch/3
  Switch/1 -> Demux/1
  Demux/1 -> Subsystem3/1(T1), Add2/1
  Demux/2 -> Add2/2, Subsystem3/3(T2)
  VoltReconstruct/1(Uanbncn) -> Scope2/1
  MATLAB Function/2(y2) -> Mux4/2
  MATLAB Function/1(y1) -> Mux4/1
  Switch1/1 -> Switch/1
  Constant1/1 -> Switch1/2
  Mux4/1 -> Switch1/1
  MATLAB Function1/2(y2) -> Add1/2, Mux5/2
  MATLAB Function1/1(y1) -> Add1/1, Mux5/1
  Mux2/1 -> Manual Switch/1
  Mux5/1 -> Manual Switch/2
  Manual Switch/1 -> Switch1/3
  Add/1 -> Mux6/2
  Add1/1 -> Mux7/2
  Mux6/1 -> Scope3/1
  Mux7/1 -> Scope3/2
  T/1 -> Mux7/1, Subsystem6/2(T), MATLAB Function2/3(Ts), Mux8/1, Mux6/1, MATLAB Function1/3(Ts), MATLAB Function/3(Ts), Subsystem3/2(T), Subsystem1/1(T)
  Mux8/1 -> Scope3/3
  Add2/1 -> Mux8/2
  MATLAB Function2/2(y2) -> Subsystem6/3(T2)
  Subsystem6/1(Ta) -> Mux9/1
  Subsystem6/3(Tc) -> Mux9/3
  Subsystem6/2(Tb) -> Mux9/2
  Mux9/1 -> Gain3/1
  Gain3/1 -> Demux2/1
  Demux1/2 -> Mux10/1  "1"
  Demux2/2 -> Mux10/2  "2"
  Mux10/1 -> Scope4/1
  Demux1/1 -> Mux11/1
  Demux2/1 -> Mux11/2
  Mux11/1 -> Scope5/1
  Demux2/3 -> Mux12/2
  Demux1/3 -> Mux12/1
  Mux12/1 -> Scope6/1
  MATLAB Function2/1(y1) -> Subsystem6/1(T1)
  VoltReconstruct/2(Uaoboco) -> Scope2/2
  Constant2/1 -> Add3/1
  Mux13/1 -> Add3/2
  Add3/1 -> Gain4/1
  Gain4/1 -> Gain5/1, Scope7/1
  Gain5/1 -> Scope8/1

== system FluxModel2015a_verify_Q_zhixin/Signal Builder ==
  Demux : Demux  Tag=STV Demux  Outputs=1
      settings: DisplayOption=none
  FromWs : FromWorkspace  Tag=STV FromWs  VariableName=tuvar
      SigBuilderData=|
      | common.afterFinalStr = 'Extrapolate'
      | common.sampleTime = 0
      | dataSet.timeRange = [0 10]
      | dataSet.name = 'Group 1'
      | sbobj.Groups.Name = 'Group 1'
      | sbobj.Groups.Signals.Name = 'Signal 2'
      | sbobj.Groups.Signals.XData = [0 5 5 10]
      | sbobj.Groups.Signals.YData = [0 1 1 0]
  Signal 2 : Outport  Tag=STV Outport
  wires:
  FromWs/1 -> Demux/1
  Demux/1 -> Signal 2/1

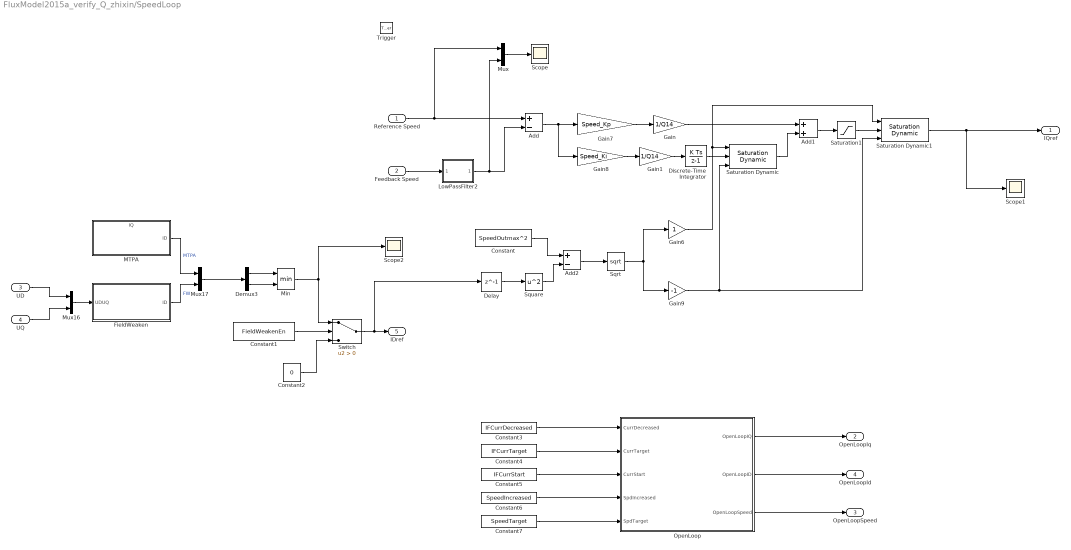
== system FluxModel2015a_verify_Q_zhixin/SpeedLoop ==
  Reference Speed : Inport
  Feedback Speed : Inport  Port=2
  UD : Inport  Port=3
  UQ : Inport  Port=4
  Trigger : TriggerPort  VariantControl=Variant  PortDimensions=1
  Add : Sum  Inputs=+-
  Add1 : Sum
  Add2 : Sum  Inputs=+-
  Constant : Constant  Value=SpeedOutmax^2
  Constant1 : Constant  Value=FieldWeakenEn
  Constant2 : Constant  Value=0
  Constant3 : Constant  Value=IFCurrDecreased
  Constant4 : Constant  Value=IFCurrTarget
  Constant5 : Constant  Value=IFCurrStart
  Constant6 : Constant  Value=SpeedIncreased
  Constant7 : Constant  Value=SpeedTarget
  Delay : Delay  DelayLength=1
  Demux3 : Demux  Outputs=2
  Discrete-Time Integrator : DiscreteIntegrator  gainval=1.0/tb  SampleTime=-1  LimitOutput=on  UpperSaturationLimit=SpeedOutmax  LowerSaturationLimit=-SpeedOutmax  ICPrevOutput=DiscIntNeverNeededParam  ICPrevScaledInput=DiscIntNeverNeededParam
  FieldWeaken : Subsystem
  Gain : Gain  Gain=1/Q14
  Gain1 : Gain  Gain=1/Q14
  Gain6 : Gain
  Gain7 : Gain  Gain=Speed_Kp
  Gain8 : Gain  Gain=Speed_Ki
  Gain9 : Gain  Gain=-1
  LowPassFilter2 : Subsystem
  MTPA : Subsystem
      settings: PortSchema="{\"entries\":[{\"content\":{\"sides\":[{\"content\":{\"connectorIds\":[]},\"type\":\"ConnectorPlacement.EquallySpacedRectSide\",\"uuid\":\"a5904245-4ea6-4d6d-a524-a9289c0225a6\"},{\"content\":{\"connectorIds\":[\"Out1\"],\"side\":\"RIGHT\"},\"type\":\"ConnectorPlacement.EquallySpacedRectSide\",\"uuid\":\"60983ff3-a156-4868-be5e-bf62d665d4eb\"},{\"content\":{\"connectorIds\":[\"In1\"],\"side\":\"TOP\"},\"type\":\"ConnectorPlacement.EquallySpacedRectSide\",\"uuid\":\"474b3f1b-69f7-4d3b-95eb-2704c9a64f09\"},{\"content\":{\"connectorIds\":[],\"side\":\"HIDDEN\"},\"type\":\"ConnectorPlacement.EquallySpacedRectSide\",\"uuid\":\"4d5a81f1-6675-4864-8749-0d48e39305a2\"}]},\"type\":\"ConnectorPlacement.EquallySpacedConnector\",\"uuid\":\"566d7f91-92d4-4d90-8232-38b94aeb0503\"}],\"packageUris\":[\"http://schema.mathworks.com/mf0/Connector/R2020b\"],\"version\":\"1.0\"}"
  Min : MinMax  Inputs=2
  Mux : Mux  Inputs=2
  Mux16 : Mux  Inputs=2
  Mux17 : Mux  Inputs=2
  OpenLoop : Subsystem
  Saturation Dynamic : simulink/Discontinuities/Saturation Dynamic  OutMin=[]  OutMax=[]  OutDataTypeStr=Inherit: Same as second input  OutDataType=fixdt(1, 16)  OutScaling=2^-10  DoSatur=off
  Saturation Dynamic1 : simulink/Discontinuities/Saturation Dynamic  OutMin=[]  OutMax=[]  OutDataTypeStr=Inherit: Same as second input  OutDataType=fixdt(1, 16)  OutScaling=2^-10  DoSatur=off
  Saturation1 : Saturate  UpperLimit=SpeedOutmax  LowerLimit=-SpeedOutmax
  Scope : Scope
  Scope1 : Scope
  Scope2 : Scope
  Sqrt : Sqrt  SaturateOnIntegerOverflow=on
  Square : Math  Operator=square  SaturateOnIntegerOverflow=on
  Switch : Switch  Criteria=u2 > Threshold
  IQref : Outport
  OpenLoopIq : Outport  Port=2
  OpenLoopSpeed : Outport  Port=3
  OpenLoopId : Outport  Port=4
  IDref : Outport  Port=5
  wires:
  Add/1 -> Gain7/1, Gain8/1
  Gain9/1 -> Saturation Dynamic1/3, Saturation Dynamic/3
  Discrete-Time Integrator/1 -> Saturation Dynamic/2
  FieldWeaken/1(ID) -> Mux17/2  "FW"
  Add2/1 -> Sqrt/1
  Square/1 -> Add2/2
  Gain6/1 -> Saturation Dynamic1/1, Saturation Dynamic/1
  Delay/1 -> Square/1
  Demux3/2 -> Min/2
  Add1/1 -> Saturation1/1
  UD/1 -> Mux16/1
  Saturation Dynamic/1 -> Add1/2
  UQ/1 -> Mux16/2
  Constant/1 -> Add2/1
  Sqrt/1 -> Gain9/1, Gain6/1
  Mux16/1 -> FieldWeaken/1(UDUQ)
  Mux17/1 -> Demux3/1
  MTPA/1(ID) -> Mux17/1  "MTPA"
  Reference Speed/1 -> Mux/1, Add/1
  Demux3/1 -> Min/1
  OpenLoop/1(OpenLoopIQ) -> OpenLoopIq/1
  Constant3/1 -> OpenLoop/1(CurrDecreased)
  Constant5/1 -> OpenLoop/3(CurrStart)
  OpenLoop/3(OpenLoopSpeed) -> OpenLoopSpeed/1
  Constant7/1 -> OpenLoop/5(SpdTarget)
  Constant6/1 -> OpenLoop/4(SpdIncreased)
  Constant4/1 -> OpenLoop/2(CurrTarget)
  OpenLoop/2(OpenLoopID) -> OpenLoopId/1
  Mux/1 -> Scope/1
  Gain7/1 -> Gain/1
  Gain8/1 -> Gain1/1
  Min/1 -> Switch/1, Scope2/1
  Saturation Dynamic1/1 -> Scope1/1, IQref/1
  Saturation1/1 -> Saturation Dynamic1/2
  Gain/1 -> Add1/1
  Gain1/1 -> Discrete-Time Integrator/1
  Constant1/1 -> Switch/2
  Switch/1 -> Delay/1, IDref/1
  Constant2/1 -> Switch/3
  Feedback Speed/1 -> LowPassFilter2/1(Input)
  LowPassFilter2/1(Output) -> Mux/2, Add/2

== system FluxModel2015a_verify_Q_zhixin/Subsystem ==
  RPM_realtime : Inport
  Gain14 : Gain  Gain=Tn/(Speedn^2)
  Math Function : Math  Operator=square  SaturateOnIntegerOverflow=on
  Product : Product
  Sign : Signum
  torque : Outport
  wires:
  RPM_realtime/1 -> Sign/1, Math Function/1
  Math Function/1 -> Gain14/1
  Gain14/1 -> Product/2
  Product/1 -> torque/1
  Sign/1 -> Product/1

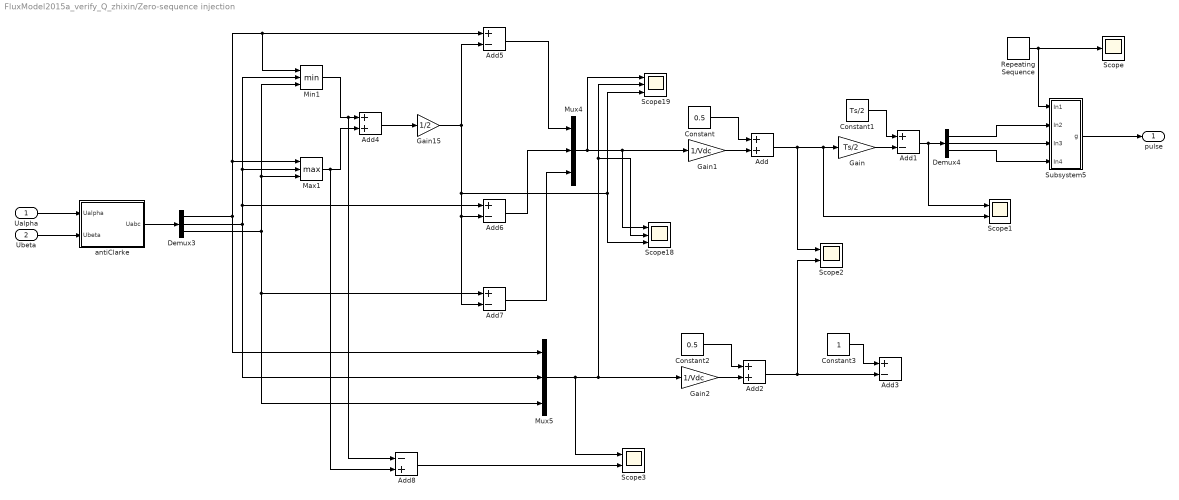
== system FluxModel2015a_verify_Q_zhixin/Zero-sequence injection ==
  Ualpha : Inport
  Ubeta : Inport  Port=2
  Add : Sum
  Add{1,3,5..7} (5 alike) : Sum  Inputs=+-
  Add2 : Sum
  Add4 : Sum
  Add8 : Sum  Inputs=-+
  Constant : Constant  Value=0.5
  Constant1 : Constant  Value=Ts/2
  Constant2 : Constant  Value=0.5
  Constant3 : Constant
  Demux3 : Demux  Outputs=3
  Demux4 : Demux  Outputs=3
  Gain : Gain  Gain=Ts/2
  Gain1 : Gain  Gain=1/Vdc
  Gain15 : Gain  Gain=1/2
  Gain2 : Gain  Gain=1/Vdc
  Max1 : MinMax  Function=max  Inputs=3
  Min1 : MinMax  Inputs=3
  Mux4 : Mux  Inputs=3
  Mux5 : Mux  Inputs=3
  Repeating Sequence : simulink/Sources/Repeating Sequence  rep_seq_t=[0 Ts/2 Ts]  rep_seq_y=[0 Ts/2 0]
  Scope : Scope
  Scope1 : Scope  NumInputPorts=2
  Scope18 : Scope  NumInputPorts=3
  Scope19 : Scope  NumInputPorts=3
  Scope2 : Scope  NumInputPorts=2
  Scope3 : Scope  NumInputPorts=2
  Subsystem5 : Subsystem
  antiClarke : Subsystem
  pulse : Outport
  wires:
  Demux3/3 -> Max1/3, Min1/3, Add7/1, Mux5/3
  Add6/1 -> Mux4/2
  Subsystem5/1(g) -> pulse/1
  Demux3/1 -> Add5/1, Min1/1, Max1/1, Mux5/1
  Add4/1 -> Gain15/1
  Max1/1 -> Add8/2, Add4/2
  Demux4/3 -> Subsystem5/4(In4)
  Ualpha/1 -> antiClarke/1(Ualpha)
  Mux5/1 -> Scope3/1, Gain2/1, Scope19/2, Scope18/2
  Add5/1 -> Mux4/1
  Gain15/1 -> Scope18/3, Scope19/3, Add7/2, Add6/2, Add5/2
  Min1/1 -> Add8/1, Add4/1
  Demux4/2 -> Subsystem5/3(In3)
  Demux4/1 -> Subsystem5/2(In2)
  Repeating Sequence/1 -> Scope/1, Subsystem5/1(In1)
  Demux3/2 -> Min1/2, Max1/2, Add6/1, Mux5/2
  Add7/1 -> Mux4/3
  antiClarke/1(Uabc) -> Demux3/1
  Ubeta/1 -> antiClarke/2(Ubeta)
  Mux4/1 -> Gain1/1, Scope18/1, Scope19/1
  Gain1/1 -> Add/2
  Constant/1 -> Add/1
  Add/1 -> Gain/1, Scope1/2, Scope2/1
  Constant2/1 -> Add2/1
  Add2/1 -> Scope2/2, Add3/2
  Constant3/1 -> Add3/1
  Gain2/1 -> Add2/2
  Gain/1 -> Add1/2
  Constant1/1 -> Add1/1
  Add1/1 -> Scope1/1, Demux4/1
  Add8/1 -> Scope3/2

== system FluxModel2015a_verify_Q_zhixin/ZeroSeq_Inject_Example ==
  In1 : Inport
  In2 : Inport  Port=2
  In3 : Inport  Port=3
  Add : Sum
  Add1 : Sum  Inputs=+-
  Add2 : Sum  Inputs=+-
  Add3 : Sum  Inputs=+-
  Gain14 : Gain  Gain=1/2
  Max : MinMax  Function=max  Inputs=3
  Min : MinMax  Inputs=3
  Mux2 : Mux  Inputs=3
  Mux3 : Mux  Inputs=3
  Scope16 : Scope  NumInputPorts=3
  Scope17 : Scope  NumInputPorts=3
  wires:
  Min/1 -> Add/1
  Gain14/1 -> Scope17/3, Scope16/3, Add3/2, Add2/2, Add1/2
  In3/1 -> Mux3/3, Add3/1, Max/3, Min/3
  Mux3/1 -> Scope17/2, Scope16/2
  In2/1 -> Mux3/2, Add2/1, Max/2, Min/2
  Mux2/1 -> Scope16/1, Scope17/1
  In1/1 -> Mux3/1, Max/1, Add1/1, Min/1
  Add3/1 -> Mux2/3
  Add1/1 -> Mux2/1
  Max/1 -> Add/2
  Add2/1 -> Mux2/2
  Add/1 -> Gain14/1

== system FluxModel2015a_verify_Q_zhixin/CurrLoop&Observer/GivenAngle ==
  Speed : Inport
  Discrete-Time Integrator : DiscreteIntegrator  gainval=1.0/tb  SampleTime=-1  ICPrevOutput=DiscIntNeverNeededParam  ICPrevScaledInput=DiscIntNeverNeededParam
  Fcn1 : Fcn  Expr=rem((u(1)),(2*pi))
  Fcn2 : Fcn  Expr=rem((u(1)),(65535))
  Gain : Gain  Gain=10430
  Gain1 : Gain  Gain=(2*pi)/65535
  Mux : Mux  Inputs=3
  Mux1 : Mux  Inputs=2
  Scope : Scope
  Scope1 : Scope
  Angle : Outport
  wires:
  Fcn2/1 -> Mux1/1, Mux/2, Gain1/1
  Speed/1 -> Discrete-Time Integrator/1
  Discrete-Time Integrator/1 -> Fcn1/1, Gain/1
  Gain/1 -> Mux/3, Fcn2/1
  Gain1/1 -> Mux/1, Angle/1
  Mux/1 -> Scope/1
  Fcn1/1 -> Mux1/2
  Mux1/1 -> Scope1/1

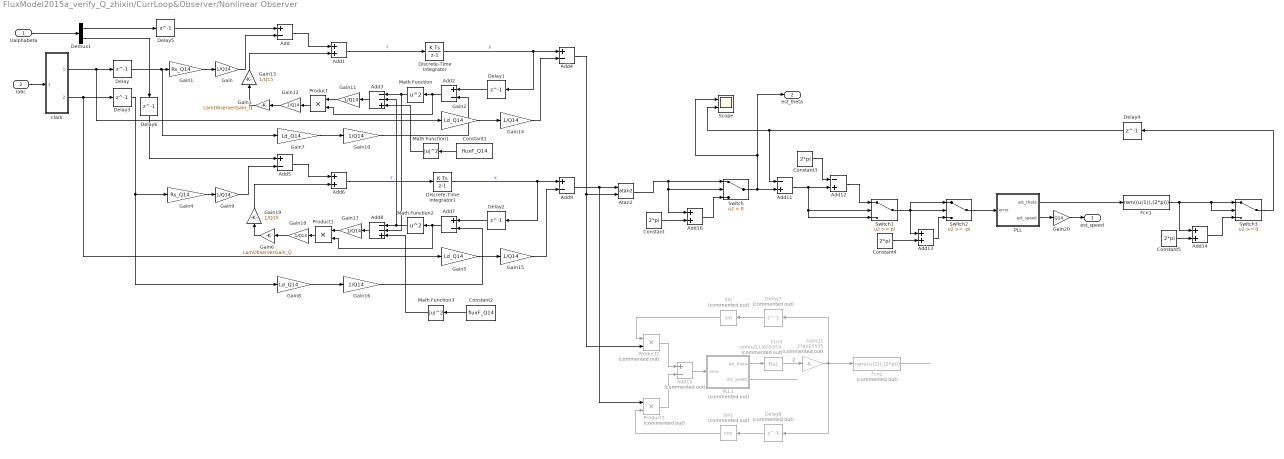
== system FluxModel2015a_verify_Q_zhixin/CurrLoop&Observer/Nonlinear Observer ==
  Ualphabeta : Inport
  Iabc : Inport  Port=2
  Add{,2,4..5,7,9} (6 alike) : Sum  Inputs=+-
  Add{1,6,10,13..14} (5 alike) : Sum
  Add11 : Sum  Inputs=-+
  Add12 : Sum  Inputs=-+
  Add15 : Sum  Commented=on  Inputs=+-
  Add3 : Sum  Inputs=--+
  Add8 : Sum  Inputs=--+
  Atan2 : Trigonometry  Operator=atan2
  Constant{,3..5} (4 alike) : Constant  Value=2*pi
  Constant1 : Constant  Value=fluxF_Q14
  Constant2 : Constant  Value=fluxF_Q14
  Delay{,1..6} (7 alike) : Delay  DelayLength=1
  Delay7 : Delay  Commented=on  DelayLength=1
  Delay8 : Delay  Commented=on  DelayLength=1
  Demux1 : Demux  Outputs=2
  Discrete-Time Integrator : DiscreteIntegrator  gainval=1.0/tb  InitialCondition=fluxF_Q14  SampleTime=-1  ICPrevOutput=DiscIntNeverNeededParam  ICPrevScaledInput=DiscIntNeverNeededParam
  Discrete-Time Integrator1 : DiscreteIntegrator  gainval=1.0/tb  InitialCondition=fluxF_Q14  SampleTime=-1  ICPrevOutput=DiscIntNeverNeededParam  ICPrevScaledInput=DiscIntNeverNeededParam
  Fcn1 : Fcn  Expr=rem((u(1)),(2*pi))
  Fcn2 : Fcn  Commented=on  Expr=rem((u(1)),(2*pi))
  Fcn3 : Fcn  Commented=on  Expr=rem(u(1),(65535))
  Gain{,9..12,14..18} (10 alike) : Gain  Gain=1/Q14
  Gain1 : Gain  Gain=Rs_Q14
  Gain13 : Gain  Gain=1/Q15
  Gain19 : Gain  Gain=1/Q15
  Gain{2,5,7..8} (4 alike) : Gain  Gain=Ld_Q14
  Gain20 : Gain  Gain=Q14
  Gain21 : Gain  Commented=on  Gain=2*pi/65535
  Gain3 : Gain  Gain=LamObserverGain_Q
  Gain4 : Gain  Gain=Rs_Q14
  Gain6 : Gain  Gain=LamObserverGain_Q
  Math Function : Math  Operator=square  SaturateOnIntegerOverflow=on
  Math Function1 : Math  Operator=magnitude^2  SaturateOnIntegerOverflow=on
  Math Function2 : Math  Operator=square  SaturateOnIntegerOverflow=on
  Math Function3 : Math  Operator=magnitude^2  SaturateOnIntegerOverflow=on
  PLL : Subsystem
  PLL1 : Subsystem  Commented=on
  Product : Product
  Product1 : Product
  Product2 : Product  Commented=on
  Product3 : Product  Commented=on
  Scope : Scope  NumInputPorts=2
  Sin : Trigonometry  Commented=on
  Sin1 : Trigonometry  Commented=on  Operator=cos
  Switch : Switch  Criteria=u2 > Threshold
  Switch1 : Switch  Threshold=pi
  Switch2 : Switch  Threshold=-pi
  Switch3 : Switch
  clark : Subsystem
  est_speed : Outport
  est_theta : Outport  Port=2
  wires:
  Constant2/1 -> Math Function3/1
  Math Function2/1 -> Add3/2, Add8/1
  Iabc/1 -> clark/1(Iabc)
  Add7/1 -> Math Function2/1, Product1/2
  Add1/1 -> Discrete-Time Integrator/1  "Y"
  Math Function3/1 -> Add8/3
  Demux1/2 -> Delay6/1
  Gain1/1 -> Gain/1
  Delay2/1 -> Add7/1
  Math Function/1 -> Add3/1, Add8/2
  Discrete-Time Integrator1/1 -> Delay2/1, Add9/1  "X"
  Gain6/1 -> Gain19/1
  Demux1/1 -> Delay5/1
  Add2/1 -> Product/2, Math Function/1
  Add6/1 -> Discrete-Time Integrator1/1  "Y"
  Delay1/1 -> Add2/1
  Discrete-Time Integrator/1 -> Add4/1, Delay1/1  "X"
  Add5/1 -> Add6/1
  Gain4/1 -> Gain9/1
  clark/1(Ialpha) -> Gain2/1, Delay/1
  Add/1 -> Add1/1
  Gain2/1 -> Gain14/1
  Constant1/1 -> Math Function1/1
  Gain3/1 -> Gain13/1
  Math Function1/1 -> Add3/3
  clark/2(Ibeta) -> Delay3/1, Gain5/1
  Ualphabeta/1 -> Demux1/1
  Delay/1 -> Gain7/1, Gain1/1
  Delay3/1 -> Gain8/1, Gain4/1
  Atan2/1 -> Switch/1, Add10/1, Switch/2
  Add10/1 -> Switch/3
  Constant/1 -> Add10/2
  Switch/1 -> est_theta/1, Scope/1, Add11/2
  Add11/1 -> Switch1/3, Switch1/2, Add12/2
  Constant3/1 -> Add12/1
  Add12/1 -> Switch1/1
  Switch1/1 -> Switch2/1, Add13/1, Switch2/2
  Add13/1 -> Switch2/3
  Constant4/1 -> Add13/2
  Switch2/1 -> PLL/1(error)
  PLL/2(est_speed) -> Gain20/1
  Fcn1/1 -> Add14/1, Switch3/2, Switch3/1
  Add14/1 -> Switch3/3
  Constant5/1 -> Add14/2
  Switch3/1 -> Delay4/1
  Delay4/1 -> Add11/1, Scope/2
  Delay5/1 -> Add/1
  Delay6/1 -> Add5/1
  Gain5/1 -> Gain15/1
  Gain7/1 -> Gain10/1
  Gain8/1 -> Gain16/1
  Gain/1 -> Add/2
  Gain9/1 -> Add5/2
  Gain10/1 -> Add2/2
  Add3/1 -> Gain11/1
  Gain11/1 -> Product/1
  Gain12/1 -> Gain3/1
  Product/1 -> Gain12/1
  Gain13/1 -> Add1/2
  Gain14/1 -> Add4/2
  Gain15/1 -> Add9/2
  Gain16/1 -> Add7/2
  Add8/1 -> Gain17/1
  Gain17/1 -> Product1/1
  Product1/1 -> Gain18/1
  Gain18/1 -> Gain6/1
  Gain19/1 -> Add6/2
  PLL/1(est_theta) -> Fcn1/1
  Delay7/1 -> Sin/1
  PLL1/1(est_theta) -> Fcn3/1
  Sin/1 -> Product2/1
  Add4/1 -> Product2/2, Atan2/2
  Product2/1 -> Add15/1
  Add15/1 -> PLL1/1(error)
  Add9/1 -> Product3/1, Atan2/1
  Product3/1 -> Add15/2
  Delay8/1 -> Sin1/1
  Sin1/1 -> Product3/2
  Gain21/1 -> Fcn2/1, Delay7/1, Delay8/1
  PLL1/2(est_speed) -> ?
  Fcn2/1 -> ?
  Fcn3/1 -> Gain21/1  "2"
  Gain20/1 -> est_speed/1
